simulink model "Flowchart7"  (Simulink 6.0)
settings: Solver=ode45  StartTime=0.0  StopTime=10.0  RelTol=1e-3
settings Model: Creator=scaife  LastModifiedBy=scaife  ExtModeAutoUpdateStatusClock=off
settings DataIOCC: SignalLoggingName=sigsOut
settings DebuggingCC: SolverPrmCheckMsg=none
settings HardwareCC: TargetUnknown=on
settings GRTTargetCC: ModelReferenceCompliant=off  MatFileLogging=off

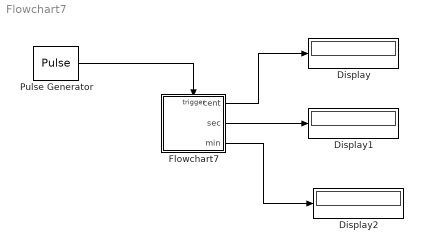
== system Flowchart7 ==
  Display : Display
  Display1 : Display
  Display2 : Display
  Flowchart7 : Stateflow chart
  Pulse Generator : DiscretePulseGenerator
  wires:
  Pulse Generator/1 -> Flowchart7/Trigger
  Flowchart7/1(cent) -> Display/1
  Flowchart7/2(sec) -> Display1/1
  Flowchart7/3(min) -> Display2/1

== stateflow chart Flowchart7 ==
  (junction 4) -> (junction 5) : [sec==3]{sec=0; min++}
  (default) -> (junction 3) : TIC{cent++}
  (junction 3) -> (junction 4) : [cent==2]{cent=0; sec++}
  (junction 3) -> (junction 5)
  (junction 4) -> (junction 5)
  data: cent output int32; sec output int32; min output int32
  events: TIC input EITHER_EDGE_EVENT
